simulink model "IP_LQG_PCI6221_2015a"  (R2015a)
settings: Solver=ode45  StartTime=0.0  StopTime=200  RelTol=1e-3
undefined symbols (not defined in the file): A_aug, ALPHA_MAX, B_aug, BETA_MAX, C_aug, K, L_aug, National_Instruments, PCI, TIME_DELAY, Ts, V_MAX, V_MIN
libraries: sldrtlib x3, simulink x2
settings Model: SimulationMode=external  CovHtmlReporting=off  ExtModeTrigDuration=100000  Creator=Alunos  LastModifiedBy=Tomas Teixeira
settings HardwareCC: ProdIntDivRoundTo=Zero  ProdEndianess=LittleEndian  ProdHWDeviceType=Intel->x86/Pentium  TargetIntDivRoundTo=Zero  TargetEndianess=LittleEndian  TargetHWDeviceType=Intel->x86/Pentium
settings RTWCC: SystemTargetFile=rtwin.tlc  TemplateMakefile=rtwin.tmf  Description=Simulink Desktop Real-Time  RTWCompilerOptimization=on
settings CodeAppCC: MaxIdLength=95
settings GRTTargetCC: TargetLangStandard=C99 (ISO)  ModelReferenceCompliant=off  ParMdlRefBuildCompliant=off  CompOptLevelCompliant=off  ConcurrentExecutionCompliant=off  CombineOutputUpdateFcns=off  MatFileLogging=off  MATLABClassNameForMDSCustomization=Simulink.SoftwareTarget.TargetSpecificTriggerConfigurationBase  CPPClassGenCompliant=off  GRTInterface=on
settings RTWinTargetCC: TargetPreCompLibLocation=C:\Program Files\MATLAB\R2015a\toolbox\sldrt\lib\win32

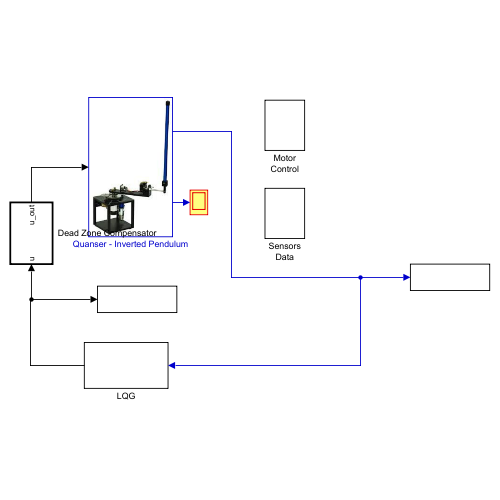
[thumbnail: Simulink's stored preview of the top-level diagram]
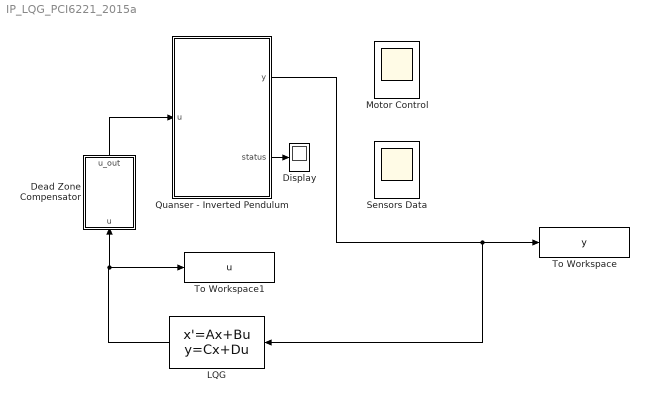
== system IP_LQG_PCI6221_2015a ==
  Dead Zone Compensator : MATLAB Function  TreatAsAtomicUnit=on
      settings: PermitHierarchicalResolution=ParametersOnly
  Display : Display
  LQG : StateSpace  A=A_aug - B_aug * K - L_aug * C_aug  B=L_aug  C=-K  D=zeros(1,2)  X0=zeros(6,1)
  Motor Control : Scope
      settings: Floating=on  TimeRange=Auto  ShowLegends=on  MaxDataPoints=5000  SaveToWorkspace=off  SaveName=ScopeData2  YMin=-10  YMax=10  SampleTime=-1
  Quanser - Inverted Pendulum : Subsystem
      mask Display: image('IP_QUANSER.jpg');
  Sensors Data : Scope
      settings: Floating=on  TimeRange=Auto  ShowLegends=on  MaxDataPoints=5000  SaveToWorkspace=off  YMin=-3.1915926535897929  YMax=3.1915926535897929  SampleTime=-1
  To Workspace : ToWorkspace  VariableName=y  SampleTime=-1
  To Workspace1 : ToWorkspace  VariableName=u  SampleTime=-1
  wires:
  Quanser - Inverted Pendulum/1(y) -> LQG/1, To Workspace/1
  Quanser - Inverted Pendulum/2(status) -> Display/1
  LQG/1 -> Dead Zone Compensator/1(u), To Workspace1/1
  Dead Zone Compensator/1(u_out) -> Quanser - Inverted Pendulum/1(u)

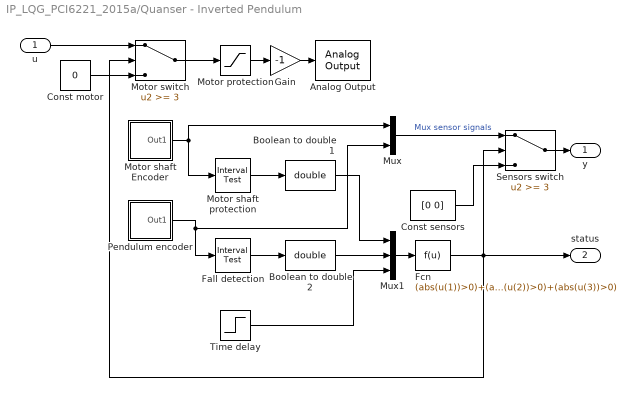
== system IP_LQG_PCI6221_2015a/Quanser - Inverted Pendulum ==
  u : Inport
  Analog Output : sldrtlib/Analog Output  SampleTime=Ts  MaxMissedTicks=10  ShowMissedTicks=off  YieldWhenWaiting=off  DrvName=National_Instruments/PCI-6221  DrvAddress=4294967295  DrvOptions=[0 0 0 2 2]  Channels=1  RangeMode=1  VoltRange=1  InitialValue=0  FinalValue=0
      settings: AttributesFormatString=National Instruments\nPCI-6221 [auto]
  Boolean to double 1 : DataTypeConversion  OutDataTypeStr=double
  Boolean to double 2 : DataTypeConversion  OutDataTypeStr=double
  Const motor : Constant  Value=0
  Const sensors : Constant  Value=[0 0]
  Fall detection : simulink/Logic and Bit Operations/Interval Test  IntervalClosedRight=on  uplimit=BETA_MAX  IntervalClosedLeft=on  lowlimit=-BETA_MAX  OutDataTypeStr=uint8
  Fcn : Fcn  Expr=(abs(u(1))>0)+(abs(u(2))>0)+(abs(u(3))>0)
  Gain : Gain  Gain=-1
  Motor protection : Saturate  UpperLimit=V_MAX  LowerLimit=V_MIN
  Motor shaft Encoder : Subsystem
  Motor shaft protection : simulink/Logic and Bit Operations/Interval Test  IntervalClosedRight=on  uplimit=ALPHA_MAX  IntervalClosedLeft=on  lowlimit=-ALPHA_MAX  OutDataTypeStr=uint8
  Motor switch : Switch  Threshold=3
  Mux : Mux  Inputs=2
  Mux1 : Mux  Inputs=3
  Pendulum encoder : Subsystem
  Sensors switch : Switch  Threshold=3
  Time delay : Step  Time=TIME_DELAY  SampleTime=0
  y : Outport
  status : Outport  Port=2
  wires:
  u/1 -> Motor switch/1
  Motor switch/1 -> Motor protection/1
  Const motor/1 -> Motor switch/3
  Motor shaft Encoder/1(Out1) -> Mux/1, Motor shaft protection/1
  Pendulum encoder/1(Out1) -> Fall detection/1, Mux/2
  Mux1/1 -> Fcn/1
  Fcn/1 -> Sensors switch/2, status/1, Motor switch/2
  Time delay/1 -> Mux1/3
  Fall detection/1 -> Boolean to double 2/1
  Boolean to double 2/1 -> Mux1/2
  Motor shaft protection/1 -> Boolean to double 1/1
  Boolean to double 1/1 -> Mux1/1
  Const sensors/1 -> Sensors switch/3
  Mux/1 -> Sensors switch/1  "Mux sensor signals"
  Sensors switch/1 -> y/1
  Gain/1 -> Analog Output/1
  Motor protection/1 -> Gain/1

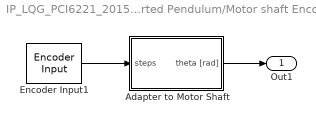
== system IP_LQG_PCI6221_2015a/Quanser - Inverted Pendulum/Motor shaft Encoder ==
  Adapter to Motor Shaft : Subsystem
  Encoder Input1 : sldrtlib/Encoder Input  SampleTime=Ts  MaxMissedTicks=inf  ShowMissedTicks=off  YieldWhenWaiting=off  DrvName=National_Instruments/PCI-6221  DrvAddress=4294967295  DrvOptions=[0 0 0 2 2]  Channels=1  QuadMode=3  IndexPulse=2  InputFilter=Inf  DataType=1
      settings: AttributesFormatString=National Instruments\nPCI-6221 [auto]
  Out1 : Outport
  wires:
  Encoder Input1/1 -> Adapter to Motor Shaft/1(steps)
  Adapter to Motor Shaft/1(theta [rad]) -> Out1/1

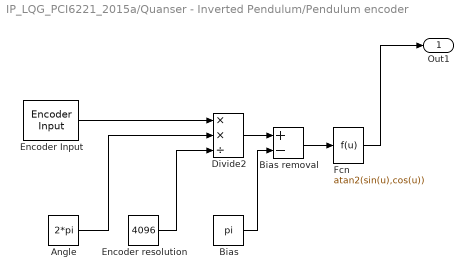
== system IP_LQG_PCI6221_2015a/Quanser - Inverted Pendulum/Pendulum encoder ==
  Angle : Constant  Value=2*pi
  Bias : Constant  Value=pi
  Bias removal : Sum  Inputs=+-
  Divide2 : Product  Inputs=**/
  Encoder resolution : Constant  Value=4096
  Encoder Input : sldrtlib/Encoder Input  SampleTime=Ts  MaxMissedTicks=inf  ShowMissedTicks=off  YieldWhenWaiting=off  DrvName=National_Instruments/PCI-6221  DrvAddress=4294967295  DrvOptions=[0 0 0 2 2]  Channels=2  QuadMode=3  IndexPulse=2  InputFilter=Inf  DataType=1
      settings: AttributesFormatString=National Instruments\nPCI-6221 [auto]
  Fcn : Fcn  Expr=atan2(sin(u),cos(u))
  Out1 : Outport
  wires:
  Bias/1 -> Bias removal/2
  Encoder resolution/1 -> Divide2/3
  Divide2/1 -> Bias removal/1
  Fcn/1 -> Out1/1
  Encoder Input/1 -> Divide2/1
  Bias removal/1 -> Fcn/1
  Angle/1 -> Divide2/2

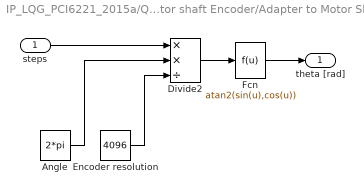
== system IP_LQG_PCI6221_2015a/Quanser - Inverted Pendulum/Motor shaft Encoder/Adapter to Motor Shaft ==
  steps : Inport
  Angle : Constant  Value=2*pi
  Divide2 : Product  Inputs=**/
  Encoder resolution : Constant  Value=4096
  Fcn : Fcn  Expr=atan2(sin(u),cos(u))
  theta [rad] : Outport
  wires:
  Angle/1 -> Divide2/2
  Encoder resolution/1 -> Divide2/3
  steps/1 -> Divide2/1
  Divide2/1 -> Fcn/1
  Fcn/1 -> theta [rad]/1

== matlab function IP_LQG_PCI6221_2015a/Dead Zone Compensator ==
  data: u input; u_out output
function u_out = fcn(u) 
    if u>0
        u_out= u + 0.2;
    elseif u<0
        u_out= u - 0.2;
    else 
        u_out = u;
    end
end
